simulink model "example2_3Leg2Level_VSC"  (R2022a)
settings: Solver=ode3  StartTime=0.0  StopTime=0.1  FixedStep=Ts  RelTol=1e-3
InitFcn:
  | Ts = 5e-6;
  | n = 2;
  | Tw = (n*pi)/(2*pi*60*33);
undefined symbols (not defined in the file or in its folder): DiscIntNeverNeededParam
libraries: spsSeriesRLCBranchLib x9, spsIGBTDiodeLib x6, spsTriangleGeneratorLib x3, spsThreePhaseVIMeasurementLib x2, spsDCVoltageSourceLib x1, spsGroundLib x1, spspowerguiLib x1
settings Model: Creator=joshua  LastModifiedBy=PSCAD_FAN
settings SolverCC: AlgebraicLoopSolver=TrustRegion
settings DataIOCC: SaveFormat=StructureWithTime  ReturnWorkspaceOutputs=off
settings DebuggingCC: UnconnectedInputMsg=warning  UnconnectedOutputMsg=warning  UnconnectedLineMsg=warning  SFMachineParentedDataDiag=warning  ArithmeticOperatorsInVariantConditions=warning
settings SFSimCC: CustomCodeUndefinedFunction=UseInterfaceOnly
settings CodeAppCC: StateflowObjectComments=on

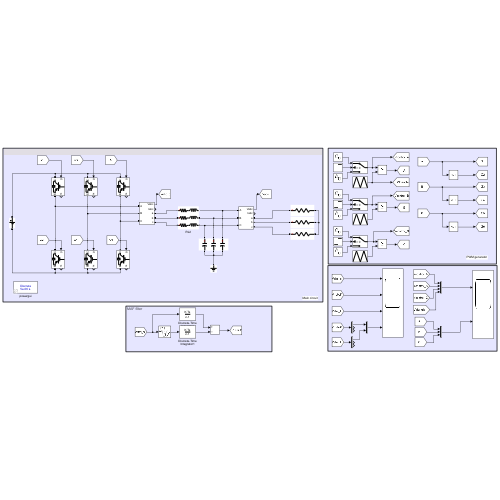
[thumbnail: Simulink's stored preview of the top-level diagram]
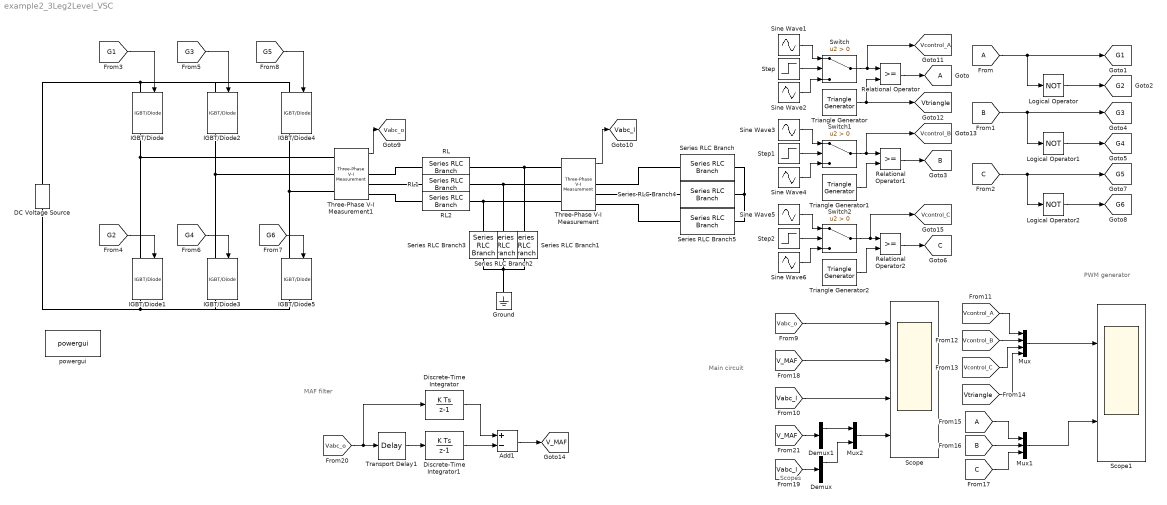
== system example2_3Leg2Level_VSC ==
  note: MAF filter
  note: Scopes
  note: PWM generator
  note: Main circuit
  Add1 : Sum  Inputs=+-
  DC Voltage Source : spsDCVoltageSourceLib/DC Voltage Source  Amplitude=200  Measurements=None
  Demux : Demux  Outputs=3
  Demux1 : Demux  Outputs=3
  Discrete-Time Integrator : DiscreteIntegrator  gainval=1/Tw  SampleTime=Ts  ICPrevOutput=DiscIntNeverNeededParam  ICPrevScaledInput=DiscIntNeverNeededParam
  Discrete-Time Integrator1 : DiscreteIntegrator  gainval=1/Tw  SampleTime=Ts  ICPrevOutput=DiscIntNeverNeededParam  ICPrevScaledInput=DiscIntNeverNeededParam
  From : From  TagVisibility=global
  From15 : From  TagVisibility=global
  Goto : Goto  TagVisibility=global
  Ground : spsGroundLib/Ground  LConnTagsString=a
  IGBT/Diode{,1..5} (6 alike) : spsIGBTDiodeLib/IGBT//Diode  Ron=1e-3  Rs=1e5  Cs=inf  Measurements=on
  Logical Operator : Logic  Operator=NOT  AllPortsSameDT=off  OutDataTypeStr=boolean
  Logical Operator1 : Logic  Operator=NOT  AllPortsSameDT=off  OutDataTypeStr=boolean
  Logical Operator2 : Logic  Operator=NOT  AllPortsSameDT=off  OutDataTypeStr=boolean
  Mux : Mux
  Mux1 : Mux  Inputs=3
  Mux2 : Mux  Inputs=2
  RL : spsSeriesRLCBranchLib/Series RLC Branch  LConnTagsString=__new0  RConnTagsString=__new0  BranchType=RL  Resistance=0.02  Inductance=3e-3  SetiL0=off  InitialCurrent=0  Capacitance=1e-6  Setx0=off  InitialVoltage=0  Measurements=None
  RL1 : spsSeriesRLCBranchLib/Series RLC Branch  LConnTagsString=__new0  RConnTagsString=__new0  BranchType=RL  Resistance=0.02  Inductance=3e-3  SetiL0=off  InitialCurrent=0  Capacitance=1e-6  Setx0=off  InitialVoltage=0  Measurements=None
  RL2 : spsSeriesRLCBranchLib/Series RLC Branch  LConnTagsString=__new0  RConnTagsString=__new0  BranchType=RL  Resistance=0.02  Inductance=3e-3  SetiL0=off  InitialCurrent=0  Capacitance=1e-6  Setx0=off  InitialVoltage=0  Measurements=None
  Relational Operator : RelationalOperator  OutDataTypeStr=boolean  InputSameDT=off
  Relational Operator1 : RelationalOperator  OutDataTypeStr=boolean  InputSameDT=off
  Relational Operator2 : RelationalOperator  OutDataTypeStr=boolean  InputSameDT=off
  Scope : Scope  NumInputPorts=4
  Scope1 : Scope  NumInputPorts=2
  Series RLC Branch : spsSeriesRLCBranchLib/Series RLC Branch  LConnTagsString=__new0  RConnTagsString=__new0  BranchType=R  Resistance=10  Inductance=1e-3  SetiL0=off  InitialCurrent=0  Capacitance=1e-6  Setx0=off  InitialVoltage=0  Measurements=None
  Series RLC Branch1 : spsSeriesRLCBranchLib/Series RLC Branch  LConnTagsString=__new0  RConnTagsString=__new0  BranchType=C  Resistance=1e-4  Inductance=200e-6  SetiL0=off  InitialCurrent=0  Capacitance=30e-6  Setx0=off  InitialVoltage=150  Measurements=None
  Series RLC Branch2 : spsSeriesRLCBranchLib/Series RLC Branch  LConnTagsString=__new0  RConnTagsString=__new0  BranchType=C  Resistance=1e-4  Inductance=200e-6  SetiL0=off  InitialCurrent=0  Capacitance=30e-6  Setx0=off  InitialVoltage=150  Measurements=None
  Series RLC Branch3 : spsSeriesRLCBranchLib/Series RLC Branch  LConnTagsString=__new0  RConnTagsString=__new0  BranchType=C  Resistance=1e-4  Inductance=200e-6  SetiL0=off  InitialCurrent=0  Capacitance=30e-6  Setx0=off  InitialVoltage=150  Measurements=None
  Series RLC Branch4 : spsSeriesRLCBranchLib/Series RLC Branch  LConnTagsString=__new0  RConnTagsString=__new0  BranchType=R  Resistance=10  Inductance=1e-3  SetiL0=off  InitialCurrent=0  Capacitance=1e-6  Setx0=off  InitialVoltage=0  Measurements=None
  Series RLC Branch5 : spsSeriesRLCBranchLib/Series RLC Branch  LConnTagsString=__new0  RConnTagsString=__new0  BranchType=R  Resistance=10  Inductance=1e-3  SetiL0=off  InitialCurrent=0  Capacitance=1e-6  Setx0=off  InitialVoltage=0  Measurements=None
  Sine Wave1 : Sin  Amplitude=0.8  Frequency=2*pi*60  SampleTime=Ts
  Sine Wave2 : Sin  Frequency=2*pi*60  SampleTime=Ts
  Sine Wave3 : Sin  Amplitude=0.8  Frequency=2*pi*60  Phase=-2*pi/3  SampleTime=Ts
  Sine Wave4 : Sin  Frequency=2*pi*60  Phase=-2*pi/3  SampleTime=Ts
  Sine Wave5 : Sin  Amplitude=0.8  Frequency=2*pi*60  Phase=2*pi/3  SampleTime=Ts
  Sine Wave6 : Sin  Frequency=2*pi*60  Phase=2*pi/3  SampleTime=Ts
  Step : Step  Time=0.05  SampleTime=Ts
  Step1 : Step  Time=0.05  SampleTime=Ts
  Step2 : Step  Time=0.05  SampleTime=Ts
  Switch : Switch  Criteria=u2 > Threshold  SaturateOnIntegerOverflow=off  InputSameDT=off
  Switch1 : Switch  Criteria=u2 > Threshold  SaturateOnIntegerOverflow=off  InputSameDT=off
  Switch2 : Switch  Criteria=u2 > Threshold  SaturateOnIntegerOverflow=off  InputSameDT=off
  Three-Phase V-I Measurement : spsThreePhaseVIMeasurementLib/Three-Phase V-I Measurement  VoltageMeasurement=phase-to-ground  SetLabelV=off  LabelV=Vabc  Vpu=off  VpuLL=off  CurrentMeasurement=yes  SetLabelI=off  LabelI=Iabc  Ipu=off  Pbase=100e6  Vbase=500e3  OutputType=Complex  PhasorSimulation=off  PSBequivalent=0
  Three-Phase V-I Measurement1 : spsThreePhaseVIMeasurementLib/Three-Phase V-I Measurement  VoltageMeasurement=phase-to-ground  SetLabelV=off  LabelV=Vabc  Vpu=off  VpuLL=off  CurrentMeasurement=yes  SetLabelI=off  LabelI=Iabc  Ipu=off  Pbase=100e6  Vbase=500e3  OutputType=Complex  PhasorSimulation=off  PSBequivalent=0
  Transport Delay1 : TransportDelay  DelayTime=Tw  PadeOrder=1
  Triangle Generator : spsTriangleGeneratorLib/Triangle Generator  Freq=60*33  Phase=0  Ts=Ts
  Triangle Generator1 : spsTriangleGeneratorLib/Triangle Generator  Freq=60*33  Phase=0  Ts=Ts
  Triangle Generator2 : spsTriangleGeneratorLib/Triangle Generator  Freq=60*33  Phase=0  Ts=Ts
  powergui : spspowerguiLib/powergui  Priority=1  SimulationMode=Discrete  SampleTime=Ts  frequency=60  Iterations=50  frequencyindice=0  Pbase=100e6  ErrMax=1e-4  UnitsV=kV  UnitsW=MW  buscounter=0  FunctionMessages=off  echomessages=off  EnableUseOfTLC=off  CurrentSourceSwitches=off  DisableSnubberDevices=off  DisableRonSwitches=off  DisableVfSwitches=off  DisplayEquations=off  AutomaticDiscreteSolvers=off  SolverType=Tustin/Backward Euler (TBE)  Interpol=off  ExternalGateDelay=off  methode=off  Ts=100  x0status=blocks  SPID=on  SwTol=0  HookPort=off  NonlinearTolerance=1e-4  nMaxIteration=100  ContinueOnMaxIteration=off  RestoreLinks=warning  ResistiveCurrentMeasurement=off  Frange=[0:2:500]  Ylog=off  Xlog=on  ShowGrid=off  save=off  variable=ZData  structure=ScopeData  ZoomFFT=off  StartTime=0.0  cycles=6  DisplayStyle=1  fundamental=60  FreqAxis=off  MaxFrequency=2000  frequencyindicesteady=1  RmsSteady=1  display=off
  tag scope: B=global, C=global, G1=global, G2=global, G3=global, G4=global, G5=global, G6=global, V_MAF=global, Vabc_l=global, Vabc_o=global, Vcontrol_A=global, Vcontrol_B=global, Vcontrol_C=global, Vtriangle=global
  wires:
  Sine Wave2/1 -> Switch/3
  From/1 -> Logical Operator/1, [G1]
  Triangle Generator/1 -> [Vtriangle], Relational Operator/2
  Switch/1 -> [Vcontrol_A], Relational Operator/1
  Logical Operator/1 -> [G2]
  Relational Operator/1 -> Goto/1
  Step/1 -> Switch/2
  Sine Wave1/1 -> Switch/1
  Sine Wave3/1 -> Switch1/1
  Step1/1 -> Switch1/2
  Relational Operator1/1 -> [B]
  Logical Operator1/1 -> [G4]
  Switch1/1 -> [Vcontrol_B], Relational Operator1/1
  Triangle Generator1/1 -> Relational Operator1/2
  [B] -> [G3], Logical Operator1/1
  Sine Wave4/1 -> Switch1/3
  Sine Wave5/1 -> Switch2/1
  Step2/1 -> Switch2/2
  Relational Operator2/1 -> [C]
  Logical Operator2/1 -> [G6]
  Switch2/1 -> [Vcontrol_C], Relational Operator2/1
  Triangle Generator2/1 -> Relational Operator2/2
  [C] -> [G5], Logical Operator2/1
  Sine Wave6/1 -> Switch2/3
  [G1] -> IGBT/Diode/1
  [G2] -> IGBT/Diode1/1
  [G3] -> IGBT/Diode2/1
  [G4] -> IGBT/Diode3/1
  [G6] -> IGBT/Diode5/1
  [G5] -> IGBT/Diode4/1
  Three-Phase V-I Measurement1/1 -> [Vabc_o]
  Three-Phase V-I Measurement/1 -> [Vabc_l]
  [Vabc_o] -> Scope/1
  [Vabc_l] -> Scope/3
  [Vcontrol_B] -> Mux/2
  [Vcontrol_A] -> Mux/1
  [Vcontrol_C] -> Mux/3
  Mux/1 -> Scope1/1
  [Vtriangle] -> Mux/4
  [B] -> Mux1/2
  From15/1 -> Mux1/1
  [C] -> Mux1/3
  Mux1/1 -> Scope1/2
  Add1/1 -> [V_MAF]
  Discrete-Time Integrator1/1 -> Add1/2
  [Vabc_o] -> Discrete-Time Integrator/1, Transport Delay1/1
  Discrete-Time Integrator/1 -> Add1/1
  Transport Delay1/1 -> Discrete-Time Integrator1/1
  [V_MAF] -> Scope/2
  [Vabc_l] -> Demux/1
  [V_MAF] -> Demux1/1
  Demux1/1 -> Mux2/1
  Demux/1 -> Mux2/2
  Mux2/1 -> Scope/4
  connections:
  DC Voltage Source/RConn1 -- IGBT/Diode2/LConn1 -- IGBT/Diode4/LConn1 -- IGBT/Diode/LConn1
  IGBT/Diode1/RConn1 -- DC Voltage Source/LConn1 -- IGBT/Diode3/RConn1 -- IGBT/Diode5/RConn1
  IGBT/Diode/RConn1 -- Three-Phase V-I Measurement1/LConn1 -- IGBT/Diode1/LConn1
  IGBT/Diode2/RConn1 -- Three-Phase V-I Measurement1/LConn2 -- IGBT/Diode3/LConn1
  IGBT/Diode4/RConn1 -- Three-Phase V-I Measurement1/LConn3 -- IGBT/Diode5/LConn1
  RL/RConn1 -- Series RLC Branch1/LConn1 -- Three-Phase V-I Measurement/LConn1
  RL1/RConn1 -- Series RLC Branch2/LConn1 -- Three-Phase V-I Measurement/LConn2
  RL2/RConn1 -- Series RLC Branch3/LConn1 -- Three-Phase V-I Measurement/LConn3
  Series RLC Branch3/RConn1 -- Series RLC Branch1/RConn1 -- Ground/LConn1 -- Series RLC Branch2/RConn1
  Series RLC Branch/RConn1 -- Series RLC Branch5/RConn1 -- Series RLC Branch4/RConn1
  Series RLC Branch/LConn1 -- Three-Phase V-I Measurement/RConn1
  Series RLC Branch4/LConn1 -- Three-Phase V-I Measurement/RConn2
  Series RLC Branch5/LConn1 -- Three-Phase V-I Measurement/RConn3
  Three-Phase V-I Measurement1/RConn2 -- RL1/LConn1
  Three-Phase V-I Measurement1/RConn1 -- RL/LConn1
  Three-Phase V-I Measurement1/RConn3 -- RL2/LConn1
